simulink model "cable_rob"  (R2023b)
settings: Solver=VariableStepAuto  StartTime=0.0  StopTime=50  RelTol=1e-3
values from neighbouring files (symbols this model uses):
  l1n0 = norm(a(:,1) - bg(:,1))    [init.m]
  l2n0 = norm(a(:,2) - bg(:,2))    [init.m]
  l3n0 = norm(a(:,3) - bg(:,3))    [init.m]
  l4n0 = norm(a(:,4) - bg(:,4))    [init.m]
  psi0 = -0.0    (= 0)    [init.m]
  x0 = -0.2    [init.m]
  y0 = -0.2    [init.m]
libraries: slpidlib x4
settings Model: Creator=aamo  LastModifiedBy=solvno

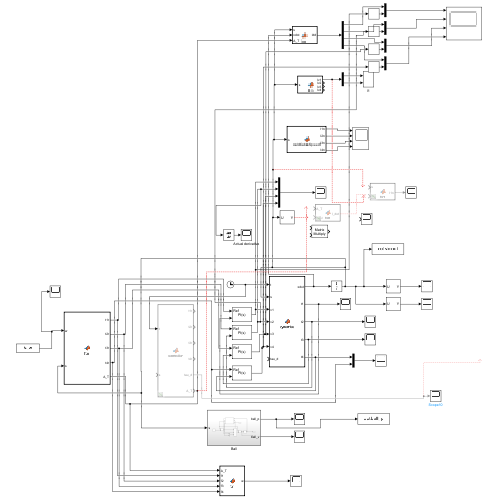
[thumbnail: Simulink's stored preview of the top-level diagram]
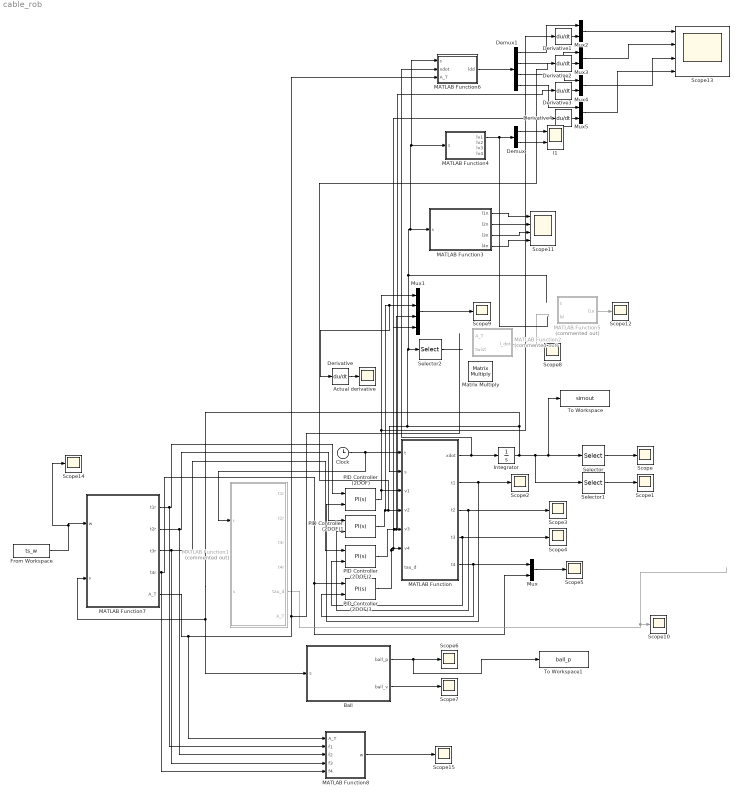
== system cable_rob ==
  Actual derivative : Scope
  Ball : Subsystem
  Clock : Clock
  Demux : Demux  Outputs=2
  Demux1 : Demux
  Derivative{,1..4} (5 alike) : Derivative
  From Workspace : FromWorkspace  VariableName=ts_w
  Integrator : Integrator  InitialCondition=[x0;y0;psi0;0;0;0;l1n0; l2n0; l3n0; l4n0]
  MATLAB Function : MATLAB Function  TreatAsAtomicUnit=on
  MATLAB Function1 : MATLAB Function  Commented=on  TreatAsAtomicUnit=on
  MATLAB Function2 : MATLAB Function  Commented=on  TreatAsAtomicUnit=on
  MATLAB Function3 : MATLAB Function  TreatAsAtomicUnit=on
  MATLAB Function4 : MATLAB Function  TreatAsAtomicUnit=on
  MATLAB Function5 : MATLAB Function  Commented=on  TreatAsAtomicUnit=on
  MATLAB Function6 : MATLAB Function  TreatAsAtomicUnit=on
  MATLAB Function7 : MATLAB Function  TreatAsAtomicUnit=on
  MATLAB Function8 : MATLAB Function  TreatAsAtomicUnit=on
  Matrix Multiply : Product  Multiplication=Matrix(*)
  Mux{,2..5} (5 alike) : Mux  Inputs=2
  Mux1 : Mux
  PID Controller (2DOF){,1..3} (4 alike) : slpidlib/PID Controller (2DOF)  Controller=PI  Form=Parallel  TimeDomain=Continuous-time  UseExternalTs=off  SampleTime=-1  IntegratorMethod=Forward Euler  FilterMethod=Forward Euler  ControllerParametersSource=internal  P=1  I=1  UseKiTs=off  D=5  N=100  UseFilter=on  b=1  c=1  TunerSelectOption=Transfer Function Based (PID Tuner App)  InitialConditionSource=internal  InitialConditionForIntegrator=0  InitialConditionForFilter=0  DifferentiatorICPrevScaledInput=0  ExternalReset=none  TrackingMode=off  Kt=1  LimitOutput=off  SatLimitsSource=internal  UpperSaturationLimit=inf  LowerSaturationLimit=-inf  LinearizeAsGain=on  AntiWindupMode=none  Kb=1  LimitIntegrator=off  UpperIntegratorSaturationLimit=inf  LowerIntegratorSaturationLimit=-inf  POutMin=[]  POutMax=[]  IOutMin=[]  IOutMax=[]  DOutMin=[]  DOutMax=[]  NOutMin=[]  NOutMax=[]  bOutMin=[]  bOutMax=[]  cOutMin=[]  cOutMax=[]  SumOutMin=[]  SumOutMax=[]  SaturationOutMin=[]  SaturationOutMax=[]  PParamMin=[]  PParamMax=[]  IParamMin=[]  IParamMax=[]  DParamMin=[]  DParamMax=[]  NParamMin=[]  NParamMax=[]  bParamMin=[]  bParamMax=[]  cParamMin=[]  cParamMax=[]  KbParamMin=[]  KbParamMax=[]  KtParamMin=[]  KtParamMax=[]  KbOutMin=[]  KbOutMax=[]  KtOutMin=[]  KtOutMax=[]  IntegratorOutMin=[]  IntegratorOutMax=[]  FilterOutMin=[]  FilterOutMax=[]  SumI1OutMin=[]  SumI1OutMax=[]  SumI2OutMin=[]  SumI2OutMax=[]  SumI3OutMin=[]  SumI3OutMax=[]  SumI4OutMin=[]  SumI4OutMax=[]  SumDOutMin=[]  SumDOutMax=[]  Sum1OutMin=[]  Sum1OutMax=[]  Sum2OutMin=[]  Sum2OutMax=[]  Sum3OutMin=[]  Sum3OutMax=[]  DifferentiatorOutMin=[]  DifferentiatorOutMax=[]  FilterDiffOutCoefMin=[]  FilterDiffOutCoefMax=[]  ReciprocalOutMin=[]  ReciprocalOutMax=[]  SumDenOutMin=[]  SumDenOutMax=[]  SumNumOutMin=[]  SumNumOutMax=[]  DivideOutMin=[]  DivideOutMax=[]  UdiffTsProdOutMin=[]  UdiffTsProdOutMax=[]  NTsProdOutMin=[]  NTsProdOutMax=[]  UintegralTsProdOutMin=[]  UintegralTsProdOutMax=[]  UngainTsProdOutMin=[]  UngainTsProdOutMax=[]  ClampingZeroOutDataTypeStr=Inherit: Inherit via back propagation  ClampingZeroOutMin=[]  ClampingZeroOutMax=[]  FilterDenConstantOutDataTypeStr=Inherit: Inherit via back propagation  FilterDenConstantOutMin=[]  FilterDenConstantOutMax=[]  PCopyOutDataTypeStr=Inherit: Inherit via back propagation  PCopyOutMin=[]  PCopyOutMax=[]  NCopyOutDataTypeStr=Inherit: Inherit via back propagation  NCopyOutMin=[]  NCopyOutMax=[]  IntegratorContinuousStateAttributes=''  IntegratorStateMustResolveToSignalObject=off  IntegratorRTWStateStorageClass=Auto  FilterContinuousStateAttributes=''  FilterStateMustResolveToSignalObject=off  FilterRTWStateStorageClass=Auto  ParallelPVariant=InternalParameters  IdealPVariant=Disabled  IVariant=InternalParameters  DVariant=Disabled  bVariant=InternalParameters  cVariant=Disabled  IntegratorVariant=Continuous  SatVariant=Disabled  AWVariant=Passthrough  PCopyVariant=Disabled  TRVariant=Disabled  FdbkBlocksVariant=Forward  IdealPFdbkVariant=Disabled  SatFdbkVariant=Disabled  DerivativeFilterVariant=Disabled  NVariant=Disabled  NCopyVariant=Disabled_SignalSpec  FilterICVariant=Disabled  IntegratorICVariant=InternalICs  ExternalResetVariant=Disabled  TRSumVariant=Passthrough  SumFdbkVariant=Disabled  SumVariant=Sum_PI  TsampFilterVariant=InternalTs  TsampNgainVariant=Passthrough  TsampIntegralVariant=Disabled_SignalSpec  ExternalSaturationOutDataTypeStr=Inherit: Same as second input
  Scope{,1..10,12,14..15} (14 alike) : Scope
  Scope11 : Scope  NumInputPorts=4
  Scope13 : Scope  NumInputPorts=4
  Selector : Selector  InputPortWidth=10  IndexOptions=Index vector (dialog)  Indices=[1 2 3]  OutputSizes=1
  Selector1 : Selector  InputPortWidth=10  IndexOptions=Index vector (dialog)  Indices=[7 8 9 10]  OutputSizes=1
  Selector2 : Selector  InputPortWidth=10  IndexOptions=Index vector (dialog)  Indices=[4 5 6]  OutputSizes=1
  To Workspace : ToWorkspace  VariableName=simout  SaveFormat=Timeseries  SampleTime=-1
  To Workspace1 : ToWorkspace  VariableName=ball_p  SaveFormat=Timeseries  SampleTime=-1
  l1 : Scope  NumInputPorts=2
  wires:
  MATLAB Function/1(xdot) -> MATLAB Function6/2(xdot), Integrator/1
  Clock/1 -> MATLAB Function1/1(t), MATLAB Function/1(t)
  Integrator/1 -> MATLAB Function7/2(s), Ball/1(s), MATLAB Function6/1(s), MATLAB Function4/1(s), MATLAB Function3/1(s), Selector2/1, MATLAB Function/2(s), Selector1/1, To Workspace/1, Selector/1
  Selector/1 -> Scope/1
  Selector1/1 -> Scope1/1
  MATLAB Function/2(t1) -> PID Controller (2DOF)/2, Scope2/1
  MATLAB Function7/1(t1r) -> MATLAB Function8/2(f1), PID Controller (2DOF)/1
  MATLAB Function7/2(t2r) -> MATLAB Function8/3(f2), PID Controller (2DOF)1/1
  MATLAB Function7/3(t3r) -> MATLAB Function8/4(f3), PID Controller (2DOF)2/1
  MATLAB Function7/4(t4r) -> MATLAB Function8/5(f4), Mux/2, PID Controller (2DOF)3/1
  MATLAB Function/3(t2) -> PID Controller (2DOF)1/2, Scope3/1
  MATLAB Function/4(t3) -> PID Controller (2DOF)2/2, Scope4/1
  MATLAB Function/5(t4) -> Mux/1, PID Controller (2DOF)3/2
  PID Controller (2DOF)1/1 -> Derivative/1, Mux1/2, Derivative2/1, MATLAB Function/4(v2)
  PID Controller (2DOF)2/1 -> Derivative3/1, Mux1/3, MATLAB Function/5(v3)
  PID Controller (2DOF)3/1 -> Mux1/4, Derivative4/1, MATLAB Function/6(v4)
  MATLAB Function1/5(tau_d) -> Scope10/1
  Mux/1 -> Scope5/1
  Ball/1(ball_p) -> To Workspace1/1, Scope6/1
  Ball/2(ball_v) -> Scope7/1
  Selector2/1 -> ?
  Mux1/1 -> Scope9/1
  MATLAB Function7/5(A_T) -> MATLAB Function8/1(A_T), MATLAB Function6/3(A_T)
  MATLAB Function2/1(l_dot) -> ?
  MATLAB Function3/1(l1n) -> Scope11/1
  MATLAB Function3/2(l2n) -> Scope11/2
  MATLAB Function3/4(l4n) -> Scope11/4
  MATLAB Function3/3(l3n) -> Scope11/3
  MATLAB Function4/1(lv1) -> Demux/1
  Demux/1 -> l1/1
  Demux/2 -> l1/2
  MATLAB Function5/1(l1n) -> Scope12/1
  PID Controller (2DOF)/1 -> Derivative1/1, Mux1/1, MATLAB Function/3(v1)
  Derivative/1 -> Actual derivative/1
  Demux1/1 -> Mux2/1
  MATLAB Function6/1(ldd) -> Demux1/1
  Demux1/4 -> Mux5/1
  Demux1/3 -> Mux4/1
  Demux1/2 -> Mux3/1
  Mux2/1 -> Scope13/1
  Mux3/1 -> Scope13/2
  Mux4/1 -> Scope13/3
  Mux5/1 -> Scope13/4
  Derivative1/1 -> Mux2/2
  Derivative2/1 -> Mux3/2
  Derivative3/1 -> Mux4/2
  Derivative4/1 -> Mux5/2
  From Workspace/1 -> Scope14/1, MATLAB Function7/1(w)
  MATLAB Function8/1(w) -> Scope15/1

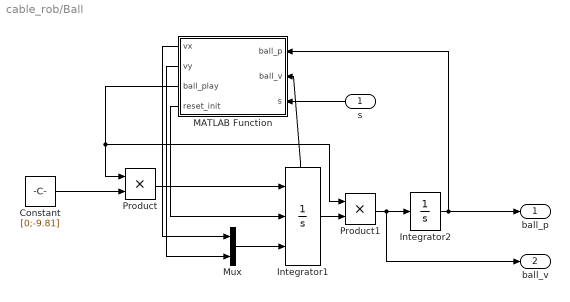
== system cable_rob/Ball ==
  s : Inport
  Constant : Constant  Value=[0;-9.81]
  Integrator1 : Integrator  ExternalReset=rising  InitialConditionSource=external  ShowStatePort=on
  Integrator2 : Integrator  InitialCondition=[0;1]
  MATLAB Function : MATLAB Function  TreatAsAtomicUnit=on
  Mux : Mux  Inputs=2
  Product : Product
  Product1 : Product
  ball_p : Outport
  ball_v : Outport  Port=2
  wires:
  Integrator2/1 -> ball_p/1, MATLAB Function/1(ball_p)
  Integrator1/1 -> Product1/2
  Constant/1 -> Product/2
  MATLAB Function/3(ball_play) -> Product/1, Product1/1
  Product/1 -> Integrator1/1
  Integrator1/State -> MATLAB Function/2(ball_v)
  Product1/1 -> ball_v/1, Integrator2/1
  MATLAB Function/4(reset_init) -> Integrator1/2
  s/1 -> MATLAB Function/3(s)
  MATLAB Function/1(vx) -> Mux/1
  MATLAB Function/2(vy) -> Mux/2
  Mux/1 -> Integrator1/3

== matlab function cable_rob/MATLAB Function7 ==
  data: w input; t1r output; t2r output; t3r output; t4r output; s input; A_T output
function [t1r,t2r,t3r,t4r, A_T] = fcn(w,s)
length=0.4; % Horizontal length of actuator
height=0.2; % Vertical length of actuator
E = 100E9;  % Young's modulus of wire
% A = 1e-6;   % Cross sectional area of wire

% Anchor points
% a1 = [ 1;  1];
% a2 = [-1;  1];
% a3 = [-1; -1];
% a4 = [ 1; -1];

% Position and rotation of actuator
% States
x   = s(1); % x-position of actuator
y   = s(2); % y-position of actuator
psi = s(3); % rotation of actuator

% Velocities
vx = s(4);
vy = s(5);
vr = s(6);

% Body anchors
% b1 = [ length/2;  height/2];
% b2 = [-length/2;  height/2];
% b3 = [-length/2; -height/2];
% b4 = [ length/2; -height/2];

a = [-1.0 1.0  1.0 -1.0;
      1.0 1.0 -1.0 -1.0];

a1 = a(:,1);
a2 = a(:,2);
a3 = a(:,3);
a4 = a(:,4);

b = [-length/2 length/2  length/2 -length/2;  
      height/2 height/2 -height/2 -height/2];
b1 = b(:,1);
b2 = b(:,2);
b3 = b(:,3);
b4 = b(:,4);

% Body anchors in global coordinates
b1g = b_to_g([x;y],psi,b1);
b2g = b_to_g([x;y],psi,b2);
b3g = b_to_g([x;y],psi,b3);
b4g = b_to_g([x;y],psi,b4);

% Length of unstretched cable rolled out.
r1 = s(7);
r2 = s(8);
r3 = s(9);
r4 = s(10);



% Compute force directions
Fd1 = (a1 - b1g)/norm(a1 - b1g);
Fd2 = (a2 - b2g)/norm(a2 - b2g);
Fd3 = (a3 - b3g)/norm(a3 - b3g);
Fd4 = (a4 - b4g)/norm(a4 - b4g);

% Compute resultant moment
R = [cos(psi), -sin(psi); sin(psi), cos(psi)];
M1 = cross([R*b1;0],[Fd1;0]);
M2 = cross([R*b2;0],[Fd2;0]);
M3 = cross([R*b3;0],[Fd3;0]);
M4 = cross([R*b4;0],[Fd4;0]);


A = [Fd1,Fd2,Fd3,Fd4;
     M1(3), M2(3), M3(3), M4(3)];
A_T = A;

coder.extrinsic('quadprog');
coder.extrinsic('optimoptions');
options = optimoptions('quadprog','Display','off');
tr = zeros(4,1);
tr = quadprog(eye(4),-5*ones(4,1),[],[],A_T, w,10*ones(4,1),100*ones(4,1), [], options);

t1r = tr(1);
t2r = tr(2);
t3r = tr(3);
t4r = tr(4);


% y = u;

== matlab function cable_rob/MATLAB Function8 ==
  data: A_T input; w output; f1 input; f2 input; f3 input; f4 input
function w = fcn(A_T, f1,f2,f3,f4)
f = [f1;f2;f3;f4];

w = A_T*f;
% y = u;

== matlab function cable_rob/MATLAB Function1 ==
  data: t input; t1r output; s input; t2r output; t3r output; t4r output; tau_d output; A_T output
function [t1r, t2r, t3r, t4r, tau_d, A_T] = controller(t,s)

% Parameters
m = 1;      % Mass of actuator
I = 1;      % Inertia of actuator
length=0.4; % Horizontal length of actuator
height=0.2; % Vertical length of actuator
E = 100E9;  % Young's modulus of wire
% A = 1e-6;   % Cross sectional area of wire

% Anchor points
a1 = [ 1;  1];
a2 = [-1;  1];
a3 = [-1; -1];
a4 = [ 1; -1];

% Position and rotation of actuator
% States
x   = s(1); % x-position of actuator
y   = s(2); % y-position of actuator
psi = s(3); % rotation of actuator

% Velocities
vx = s(4);
vy = s(5);
vr = s(6);

% Body anchors
b1 = [ length/2;  height/2];
b2 = [-length/2;  height/2];
b3 = [-length/2; -height/2];
b4 = [ length/2; -height/2];

% Body anchors in global coordinates
b1g = b_to_g([x;y],psi,b1);
b2g = b_to_g([x;y],psi,b2);
b3g = b_to_g([x;y],psi,b3);
b4g = b_to_g([x;y],psi,b4);

% Length of unstretched cable rolled out.
r1 = s(7);
r2 = s(8);
r3 = s(9);
r4 = s(10);

% Compute tau.
x_d = 0.1*[sin(5*t);
           cos(5*t);
           0];
x_dd = 0.1*[ 5*cos(5*t);
            -5*sin(5*t);
             0];
%x_d  =[0;0;0];
%x_dd = [0;0;0];
e = [x;y;psi] - x_d; % error
e_d = [vx;vy;vr] - x_dd; 
D = 10*diag([1,1,1]);
K = 15*diag([5,5,5]);
tau_d = -D*e_d - K*e;

% Compute tenstion setpoints.
%t1r = 20+5*sin(t/4+3);
%t2r = 20+5*sin(t/4+7);
%t3r = 20-5*sin(t/4+2);
%t4r = 20-5*sin(t/4+9);



% Compute force directions
Fd1 = (a1 - b1g)/norm(a1 - b1g);
Fd2 = (a2 - b2g)/norm(a2 - b2g);
Fd3 = (a3 - b3g)/norm(a3 - b3g);
Fd4 = (a4 - b4g)/norm(a4 - b4g);

% Compute resultant moment
R = [cos(psi), -sin(psi); sin(psi), cos(psi)];
M1 = cross([R*b1;0],[Fd1;0]);
M2 = cross([R*b2;0],[Fd2;0]);
M3 = cross([R*b3;0],[Fd3;0]);
M4 = cross([R*b4;0],[Fd4;0]);


A = [Fd1,Fd2,Fd3,Fd4;
     M1(3), M2(3), M3(3), M4(3)];
A_T = A;

% tr = pinv(A)*tau_d;





% function tr = forceQP(A_T, f, f_min, f_max, f_ref, w, m)
coder.extrinsic('quadprog');
coder.extrinsic('optimoptions');
options = optimoptions('quadprog','Display','off');
tr = zeros(4,1);
tr = quadprog(eye(4),-10*ones(4,1),[],[],A_T, tau_d,1*ones(4,1),100*ones(4,1), [], options);

t1r = tr(1);
t2r = tr(2);
t3r = tr(3);
t4r = tr(4);

end

function [p_g] = b_to_g(p,psi,b)
    % p: origin of body frame in global coordinates
    % psi: rotation of body frame
    % b: point in body frame.
    % p_g: Returns position of point b in global frame.

    R = R_psi(psi); %= [cos(psi), -sin(psi);sin(psi),cos(psi)];
    p_g = p + R*b;
end
function R = R_psi(psi)
    R = [cos(psi), -sin(psi);sin(psi),cos(psi)];
end

== matlab function cable_rob/MATLAB Function ==
  data: t input; xdot output; s input; t1 output; t2 output; t3 output; t4 output; v1 input; v2 input; v3 input; v4 input; tau_d input
function [xdot,t1,t2,t3,t4] = dynamics(t,s,v1,v2,v3,v4,tau_d)

% Parameters
m = 0.25;  % Mass of actuator
I = 6.25e-4; % Inertia of actuator
length=0.4; % Horizontal length of actuator
height=0.2; % Vertical length of actuator
E=100E9;    % Young's modulus of wire
A= 1e-6;    % Cross sectional area of wire

% Anchor points
% a1 = [1;1];
% a2 = [-1;1];
% a3 = [-1;-1];
% a4 = [1;-1];

% Position and rotation of actuator
% States
x = s(1); % x-position of actuator
y = s(2); % y-position of actuator
psi = s(3); % rotation of actuator

% Velocities
vx = s(4);
vy = s(5);
vr = s(6);

% Body anchors
% b1 = [ length/2;  height/2];
% b2 = [-length/2;  height/2];
% b3 = [-length/2; -height/2];
% b4 = [ length/2; -height/2];

a = [-1.0 1.0  1.0 -1.0;
      1.0 1.0 -1.0 -1.0];

a1 = a(:,1);
a2 = a(:,2);
a3 = a(:,3);
a4 = a(:,4);

b = [-length/2 length/2  length/2 -length/2;  
      height/2 height/2 -height/2 -height/2];
b1 = b(:,1);
b2 = b(:,2);
b3 = b(:,3);
b4 = b(:,4);

% Body anchors in global coordinates
b1g = b_to_g([x;y],psi,b1);
b2g = b_to_g([x;y],psi,b2);
b3g = b_to_g([x;y],psi,b3);
b4g = b_to_g([x;y],psi,b4);

% Length of unstretched cable rolled out.
r1 = s(7); 
r2 = s(8); 
r3 = s(9); 
r4 = s(10);

% Compute tensions.
t1 = A*E*(norm(b1g-a1) - r1) /r1;
t2 = A*E*(norm(b2g-a2) - r2) /r2;
t3 = A*E*(norm(b3g-a3) - r3) /r3;
t4 = A*E*(norm(b4g-a4) - r4) /r4;

% Compute forces
F1 = t1'*(a1-b1g)/norm(a1-b1g); 
F2 = t2'*(a2-b2g)/norm(a2-b2g);
F3 = t3'*(a3-b3g)/norm(a3-b3g);
F4 = t4'*(a4-b4g)/norm(a4-b4g);

% Compute resultant force
F = F1+F2+F3+F4;

% Compute resultant moment
R = [cos(psi), -sin(psi);sin(psi),cos(psi)];
M1 = cross([R*b1;0],[F1;0]);
M2 = cross([R*b2;0],[F2;0]);
M3 = cross([R*b3;0],[F3;0]);
M4 = cross([R*b4;0],[F4;0]);

% Compute resultant moment
M = M1(3)+M2(3)+M3(3)+M4(3)

xdot = [vx;vy;vr;F(1)/m;F(2)/m;M/I;-v1;-v2;-v3;-v4];

% TESTING: direct feedthrough of desired tau.
% xdot = [vx;vy;vr;tau_d(1)/m;tau_d(2)/m;tau_d(3)/I;-v1;-v2;-v3;-v4];
end

function [p_g] = b_to_g(p,psi,b)
    % p: origin of body frame in global coordinates
    % psi: rotation of body frame
    % b: point in body frame.
    % p_g: Returns position of point b in global frame.

    R = R_psi(psi); %= [cos(psi), -sin(psi);sin(psi),cos(psi)];
    p_g = p + R*b;
end
function R = R_psi(psi)
    R = [cos(psi), -sin(psi); sin(psi), cos(psi)];
end

== matlab function cable_rob/Ball/MATLAB Function ==
  data: ball_p input; vx output; vy output; ball_play output; ball_v input; reset_init output; s input
function [vx,vy,ball_play,reset_init] = fcn(ball_p,ball_v,s)

length = 0.4;
height = 0.2;

bar_p = s(1:3);
bar_v = s(4:6);

reset_init = 0;

v0 = ball_v;

if ball_p(2)<-1.2 % Ball out of bounds
    v0=[0;0];
    ball_play=0;
    reset_init = 1;
else
    ball_play=1;

    b1 = [length/2;height/2];
    b2 = [-length/2;height/2];

    % Body anchors in global coordinates
    b1g = b_to_g(s(1:2),s(3),b1);
    b2g = b_to_g(s(1:2),s(3),b2);

    if ball_p(2)<=-1
        reset_init=1;
        v0 = diag([1,-0.95])*ball_v; % Just jump off the bottom.
    elseif ball_p(1)>=b2g(1) && ball_p(1)<=b1g(1)  % Ball can potentially cross.
        dy = b1g(2)-b2g(2);
        dx = b1g(1)-b2g(1);
        inc = dy/dx;
        if ball_p(2)<=b2g(2)+inc*(ball_p(1)-b2g(1))
            reset_init=1;
            e_p = (b1g-b2g)/norm(b1g-b2g); % Paralell with bar.
            e_n = [-e_p(2);e_p(1)];        % Normal to bar.
            vip = ball_v'*e_p * e_p;
            vin = ball_v'*e_n * e_n;
            v0 = vip-vin;
        end
    end
end

vx = v0(1);
vy = v0(2);

== matlab function cable_rob/MATLAB Function2 ==
  data: A_T input; l_dot output; twist input
function l_dot = fcn(A_T,twist)
l_dot = -A_T.'*twist;
% y = u;

== matlab function cable_rob/MATLAB Function3 ==
  data: s input; l1n output; l2n output; l3n output; l4n output
function [l1n, l2n, l3n, l4n] = calcCableSpeed(s)
length=0.4; % Horizontal length of actuator
height=0.2; % Vertical length of actuator

% Anchor points
a1 = [ 1;  1];
a2 = [-1;  1];
a3 = [-1; -1];
a4 = [ 1; -1];

% Position and rotation of actuator
% States
x   = s(1); % x-position of actuator
y   = s(2); % y-position of actuator
psi = s(3); % rotation of actuator

% Velocities
vx = s(4);
vy = s(5);
vr = s(6);

% Body anchors
b1 = [ length/2;  height/2];
b2 = [-length/2;  height/2];
b3 = [-length/2; -height/2];
b4 = [ length/2; -height/2];


% l1n = 0.5*abs((2*(a1(1)-x+b1(1)*cos(psi)+b1(2)*sin(psi)) * (-vx-b1(1)*vr*sin(psi)-b1(2)*vr*cos(psi)) + 2*(a1(2)-y-b1(2)*cos(psi) + b1(1)*sin(psi))*(-vy-b1(1)*vr*cos(psi)+b1(2)*vr*sin(psi) ) )/sqrt(complex(0.5*(a1(1)-x-b1(1)*cos(psi)+b1(2)*sin(psi)))));
% l2n = 0.5*abs((2*(a2(1)-x+b2(1)*cos(psi)+b2(2)*sin(psi)) * (-vx-b2(1)*vr*sin(psi)-b2(2)*vr*cos(psi)) + 2*(a2(2)-y-b2(2)*cos(psi) + b2(1)*sin(psi))*(-vy-b2(1)*vr*cos(psi)+b2(2)*vr*sin(psi) ) )/sqrt(complex((a2(1)-x-b2(1)*cos(psi)+b2(2)*sin(psi)))));
% l3n = 0.5*abs((2*(a3(1)-x+b3(1)*cos(psi)+b3(2)*sin(psi)) * (-vx-b3(1)*vr*sin(psi)-b3(2)*vr*cos(psi)) + 2*(a3(2)-y-b3(2)*cos(psi) + b3(1)*sin(psi))*(-vy-b3(1)*vr*cos(psi)+b3(2)*vr*sin(psi) ) )/sqrt(complex((a3(1)-x-b3(1)*cos(psi)+b3(2)*sin(psi)))));
% l4n = 0.5*abs((2*(a4(1)-x+b4(1)*cos(psi)+b4(2)*sin(psi)) * (-vx-b4(1)*vr*sin(psi)-b4(2)*vr*cos(psi)) + 2*(a4(2)-y-b4(2)*cos(psi) + b4(1)*sin(psi))*(-vy-b4(1)*vr*cos(psi)+b4(2)*vr*sin(psi) ) )/sqrt(complex((a4(1)-x-b4(1)*cos(psi)+b4(2)*sin(psi)))));
l1n = (0.5)*(2*(a1(1)-x+b1(1)*cos(psi)+b1(2)*sin(psi)) * (-vx-b1(1)*vr*sin(psi)-b1(2)*vr*cos(psi)) + 2*(a1(2)-y-b1(2)*cos(psi) + b1(1)*sin(psi))*(-vy-b1(1)*vr*cos(psi)+b1(2)*vr*sin(psi) ) )/sqrt((a1(1)-x-b1(1)*cos(psi)+b1(2)*sin(psi))^2 + (a1(2) - y - b1(1)*sin(psi) - b1(2)*cos(psi))^2);
l2n = (0.5)*(2*(a2(1)-x+b2(1)*cos(psi)+b2(2)*sin(psi)) * (-vx-b2(1)*vr*sin(psi)-b2(2)*vr*cos(psi)) + 2*(a2(2)-y-b2(2)*cos(psi) + b2(1)*sin(psi))*(-vy-b2(1)*vr*cos(psi)+b2(2)*vr*sin(psi) ) )/sqrt((a2(1)-x-b2(1)*cos(psi)+b2(2)*sin(psi))^2 + (a2(2) - y - b2(1)*sin(psi) - b2(2)*cos(psi))^2);
l3n = (0.5)*(2*(a3(1)-x+b3(1)*cos(psi)+b3(2)*sin(psi)) * (-vx-b3(1)*vr*sin(psi)-b3(2)*vr*cos(psi)) + 2*(a3(2)-y-b3(2)*cos(psi) + b3(1)*sin(psi))*(-vy-b3(1)*vr*cos(psi)+b3(2)*vr*sin(psi) ) )/sqrt((a3(1)-x-b3(1)*cos(psi)+b3(2)*sin(psi))^2 + (a3(2) - y - b3(1)*sin(psi) - b3(2)*cos(psi))^2);
l4n = (0.5)*(2*(a4(1)-x+b4(1)*cos(psi)+b4(2)*sin(psi)) * (-vx-b4(1)*vr*sin(psi)-b4(2)*vr*cos(psi)) + 2*(a4(2)-y-b4(2)*cos(psi) + b4(1)*sin(psi))*(-vy-b4(1)*vr*cos(psi)+b4(2)*vr*sin(psi) ) )/sqrt((a4(1)-x-b4(1)*cos(psi)+b4(2)*sin(psi))^2 + (a4(2) - y - b4(1)*sin(psi) - b4(2)*cos(psi))^2);
% l1n = (0.5)*(2*(a1(1)-x+b1(1)*cos(psi)+b1(2)*sin(psi)) * (-vx-b1(1)*vr*sin(psi)-b1(2)*vr*cos(psi)) + 2*(a1(2)-y-b1(2)*cos(psi) + b1(1)*sin(psi))*(-vy-b1(1)*vr*cos(psi)+b1(2)*vr*sin(psi) ) )/sqrt(complex((a1(1)-x-b1(1)*cos(psi)+b1(2)*sin(psi))^2 + (a1(2) - y - b1(1)*sin(psi) - b1(2)*cos(psi))^2))
% l2n = (0.5)*(2*(a2(1)-x+b2(1)*cos(psi)+b2(2)*sin(psi)) * (-vx-b2(1)*vr*sin(psi)-b2(2)*vr*cos(psi)) + 2*(a2(2)-y-b2(2)*cos(psi) + b2(1)*sin(psi))*(-vy-b2(1)*vr*cos(psi)+b2(2)*vr*sin(psi) ) )/sqrt(complex((a2(1)-x-b2(1)*cos(psi)+b2(2)*sin(psi))^2 + (a2(2) - y - b2(1)*sin(psi) - b2(2)*cos(psi))^2))
% l3n = (0.5)*(2*(a3(1)-x+b3(1)*cos(psi)+b3(2)*sin(psi)) * (-vx-b3(1)*vr*sin(psi)-b3(2)*vr*cos(psi)) + 2*(a3(2)-y-b3(2)*cos(psi) + b3(1)*sin(psi))*(-vy-b3(1)*vr*cos(psi)+b3(2)*vr*sin(psi) ) )/sqrt(complex((a3(1)-x-b3(1)*cos(psi)+b3(2)*sin(psi))^2 + (a3(2) - y - b3(1)*sin(psi) - b3(2)*cos(psi))^2))
% l4n = (0.5)*(2*(a4(1)-x+b4(1)*cos(psi)+b4(2)*sin(psi)) * (-vx-b4(1)*vr*sin(psi)-b4(2)*vr*cos(psi)) + 2*(a4(2)-y-b4(2)*cos(psi) + b4(1)*sin(psi))*(-vy-b4(1)*vr*cos(psi)+b4(2)*vr*sin(psi) ) )/sqrt(complex((a4(1)-x-b4(1)*cos(psi)+b4(2)*sin(psi))^2 + (a4(2) - y - b4(1)*sin(psi) - b4(2)*cos(psi))^2))

% y = u;

== matlab function cable_rob/MATLAB Function4 ==
  data: s input; lv1 output; lv2 output; lv3 output; lv4 output
function [lv1, lv2, lv3, lv4] = fcn(s)
% Parameters
m = 1;      % Mass of actuator
I = 1;      % Inertia of actuator
length=0.4; % Horizontal length of actuator
height=0.2; % Vertical length of actuator
E = 100E9;  % Young's modulus of wire
% A = 1e-6;   % Cross sectional area of wire

% Anchor points
a1 = [ 1;  1];
a2 = [-1;  1];
a3 = [-1; -1];
a4 = [ 1; -1];

% Position and rotation of actuator
% States
x   = s(1); % x-position of actuator
y   = s(2); % y-position of actuator
psi = s(3); % rotation of actuator

% Velocities
vx = s(4);
vy = s(5);
vr = s(6);

% Body anchors
b1 = [ length/2;  height/2];
b2 = [-length/2;  height/2];
b3 = [-length/2; -height/2];
b4 = [ length/2; -height/2];

% Body anchors in global coordinates
b1g = b_to_g([x;y],psi,b1);
b2g = b_to_g([x;y],psi,b2);
b3g = b_to_g([x;y],psi,b3);
b4g = b_to_g([x;y],psi,b4);

% Length of unstretched cable rolled out.
r1 = s(7);
r2 = s(8);
r3 = s(9);
r4 = s(10);

% Compute tau.
% x_d = 0.1*[sin(5*t);
%            cos(5*t);
%            0];
% x_dd = 0.1*[ 5*cos(5*t);
%             -5*sin(5*t);
%              0];
%x_d  =[0;0;0];
%x_dd = [0;0;0];
% e = [x;y;psi] - x_d; % error
% e_d = [vx;vy;vr] - x_dd; 
% D = 10*diag([1,1,1]);
% K = 15*diag([5,5,5]);
% tau_d = -D*e_d - K*e;

% Compute tenstion setpoints.
%t1r = 20+5*sin(t/4+3);
%t2r = 20+5*sin(t/4+7);
%t3r = 20-5*sin(t/4+2);
%t4r = 20-5*sin(t/4+9);



% Compute force directions
lv1 = (a1 - b1g);
lv2 = (a2 - b2g);
lv3 = (a3 - b3g);
lv4 = (a4 - b4g);
% y = u;

== matlab function cable_rob/MATLAB Function5 ==
  data: s input; l1n output; ld input
function l1n = fcn(s, ld)
% Parameters
m = 1;      % Mass of actuator
I = 1;      % Inertia of actuator
length=0.4; % Horizontal length of actuator
height=0.2; % Vertical length of actuator
E = 100E9;  % Young's modulus of wire
% A = 1e-6;   % Cross sectional area of wire

% Anchor points
a1 = [ 1;  1];
a2 = [-1;  1];
a3 = [-1; -1];
a4 = [ 1; -1];

% Body anchors
b1 = [ length/2;  height/2];
b2 = [-length/2;  height/2];
b3 = [-length/2; -height/2];
b4 = [ length/2; -height/2];


bx = b1(1);
by = b1(2);

% Position and rotation of actuator
% States
x   = s(1); % x-position of actuator
y   = s(2); % y-position of actuator
psi = s(3); % rotation of actuator

% Velocities
vx = s(4);
vy = s(5);
vr = s(6);


% Body anchors in global coordinates
b1g = b_to_g([x;y],psi,b1);
b2g = b_to_g([x;y],psi,b2);
b3g = b_to_g([x;y],psi,b3);
b4g = b_to_g([x;y],psi,b4);


% Compute force directions
u1 = (a1 - b1g)/norm(a1 - b1g);
u2 = (a2 - b2g)/norm(a2 - b2g);
u3 = (a3 - b3g)/norm(a3 - b3g);
u4 = (a4 - b4g)/norm(a4 - b4g);


udbd1 = [- by*vr*cos(psi) - bx*vr*sin(psi);
        bx*vr*cos(psi) - by*vr*sin(psi)];
udbd1n = norm(udbd1,2);
% y = u;

== matlab function cable_rob/MATLAB Function6 ==
  data: s input; xdot input; ldd output; A_T input
function ldd = fcn(s, xdot, A_T)
% Parameters
m = 1;      % Mass of actuator
I = 1;      % Inertia of actuator
length=0.4; % Horizontal length of actuator
height=0.2; % Vertical length of actuator
E = 100E9;  % Young's modulus of wire
% A = 1e-6;   % Cross sectional area of wire

% Anchor points
a1 = [ 1;  1];
a2 = [-1;  1];
a3 = [-1; -1];
a4 = [ 1; -1];

% Body anchors
b1 = [ length/2;  height/2];
b2 = [-length/2;  height/2];
b3 = [-length/2; -height/2];
b4 = [ length/2; -height/2];

% Position and rotation of actuator
% States
x   = s(1); % x-position of actuator
y   = s(2); % y-position of actuator
psi = s(3); % rotation of actuator

r = [x;y];

% Velocities
vx = s(4);
vy = s(5);
vr = s(6);

rd = [vx; vy];

% Accelerations
ax = xdot(4);
ay = xdot(5);
ar = xdot(6);

rdd = [ax; ay];

% Length of unstretched cable rolled out.
l1 = s(7)
l2 = s(8);
l3 = s(9);
l4 = s(10);

twist = [vx;vy;vr];

% Norms of the derivative of cable lengths
ldn = -A_T.'*twist;
ld1n = ldn(1);
ld2n = ldn(2);
ld3n = ldn(3);
ld4n = ldn(4);

vrskew = [0, -vr; vr, 0];

arskew = [0, -ar; ar, 0];

% Body anchors in global coordinates
b1g = b_to_g([x;y],psi,b1);
b2g = b_to_g([x;y],psi,b2);
b3g = b_to_g([x;y],psi,b3);
b4g = b_to_g([x;y],psi,b4);


% Compute force directions
u1 = (a1 - b1g)/norm(a1 - b1g);
u2 = (a2 - b2g)/norm(a2 - b2g);
u3 = (a3 - b3g)/norm(a3 - b3g);
u4 = (a4 - b4g)/norm(a4 - b4g);

% u1d = -u1.'*([ax;ay] + R_p(psi)*vrskew*vrskew*b1 + R_p(psi)*arskew*b1) ...
      % - ((([x;y]-R_p(psi)*b1-a1)*ld1n^2/l1^2 - ([vx;vy]-R_p(psi)*vrskew*b1)/l1^2).' * ([vx;vy] + R_p(psi)*vrskew*b1));

l1dd = - u1.' ... % u1^T
      * (rdd + R_p(psi)*vrskew*vrskew*b1 + R_p(psi)*arskew*b1) ... % r_dd + b_i_dd
      - 1/l1^2*((r + R_p(psi)*b1-a1)*ld1n - (rd + R_p(psi)*vrskew*b1)*l1).' ... % u_d^T
      * (rd + R_p(psi)*b1); % r_d + b_i_d
l2dd = - u2.' ... % u2^T
      * (rdd + R_p(psi)*vrskew*vrskew*b2 + R_p(psi)*arskew*b2) ... % r_dd + b_i_dd
      - 1/l2^2*((r + R_p(psi)*b2-a2)*ld2n - (rd + R_p(psi)*vrskew*b2)*l2).' ... % u_d^T
      * (rd + R_p(psi)*b2); % r_d + b_i_d
l3dd = - u3.' ... % u3^T1
      * (rdd + R_p(psi)*vrskew*vrskew*b3 + R_p(psi)*arskew*b3) ... % r_dd + b_i_dd
      - 1/l3^2*((r + R_p(psi)*b3-a3)*ld3n - (rd + R_p(psi)*vrskew*b3)*l3).' ... % u_d^T
      * (rd + R_p(psi)*b3); % r_d + b_i_d
l4dd = - u4.' ... % u4^T1
      * (rdd + R_p(psi)*vrskew*vrskew*b4 + R_p(psi)*arskew*b4) ... % r_dd + b_i_dd
      - 1/l4^2*((r + R_p(psi)*b4-a4)*ld4n - (rd + R_p(psi)*vrskew*b4)*l4).' ... % u_d^T
      * (rd + R_p(psi)*b4); % r_d + b_i_d
l1dd = -1*l1dd;
l2dd = -1*l2dd;
l3dd = -1*l3dd;
l4dd = -1*l4dd;
ldd = [l1dd; l2dd; l3dd; l4dd];

end
function R = R_p(psi)
    R = [cos(psi), -sin(psi);sin(psi),cos(psi)];
end
